simulink model "practice6_2"  (Simulink 7.9)
settings: Solver=ode45  StartTime=0.0  StopTime=200  RelTol=1e-3
settings Model: Creator=sony  LastModifiedBy=sony

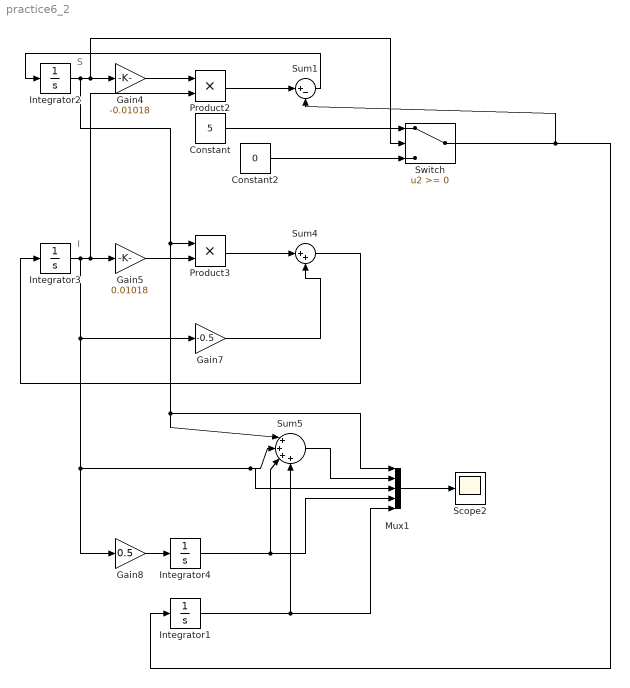
== system practice6_2 ==
  note: S
  note: I
  Constant : Constant  Value=5
  Constant2 : Constant  Value=0
  Gain4 : Gain  Gain=-0.01018
  Gain5 : Gain  Gain=0.01018
  Gain7 : Gain  Gain=-0.5
  Gain8 : Gain  Gain=0.5
  Integrator1 : Integrator
  Integrator2 : Integrator  InitialCondition=99
  Integrator3 : Integrator  InitialCondition=1
  Integrator4 : Integrator
  Mux1 : Mux  Inputs=5
  Product2 : Product  RndMeth=Zero
  Product3 : Product  RndMeth=Zero
  Scope2 : Scope
      settings: TimeRange=10
  Sum1 : Sum  Inputs=|+-
  Sum4 : Sum  Inputs=|++
  Sum5 : Sum  Inputs=|++++
  Switch : Switch
  wires:
  Integrator3/1 -> Gain5/1, Product2/2, Gain7/1, Gain8/1, Mux1/3, Sum5/2
  Integrator2/1 -> Product3/1, Sum5/1, Mux1/1, Gain4/1, Switch/2
  Gain4/1 -> Product2/1
  Gain5/1 -> Product3/2
  Product3/1 -> Sum4/1
  Gain7/1 -> Sum4/2
  Sum4/1 -> Integrator3/1
  Sum5/1 -> Mux1/2
  Mux1/1 -> Scope2/1
  Gain8/1 -> Integrator4/1
  Integrator4/1 -> Sum5/3, Mux1/4
  Integrator1/1 -> Mux1/5, Sum5/4
  Constant/1 -> Switch/1
  Constant2/1 -> Switch/3
  Product2/1 -> Sum1/1
  Switch/1 -> Sum1/2, Integrator1/1
  Sum1/1 -> Integrator2/1
